simulink model "hw3"  (R2020b)
settings: Solver=FixedStepAuto  StartTime=0.0  StopTime=6  FixedStep=0.0001  RelTol=1e-3
model workspace (MAT data in the model file):
  Analog_Amplitude = 1
  Analog_Frequncy = 1
  period = 10
libraries: dsparch4 x1
settings Model: EnablePacing=on  Creator=max  LastModifiedBy=spraychamber

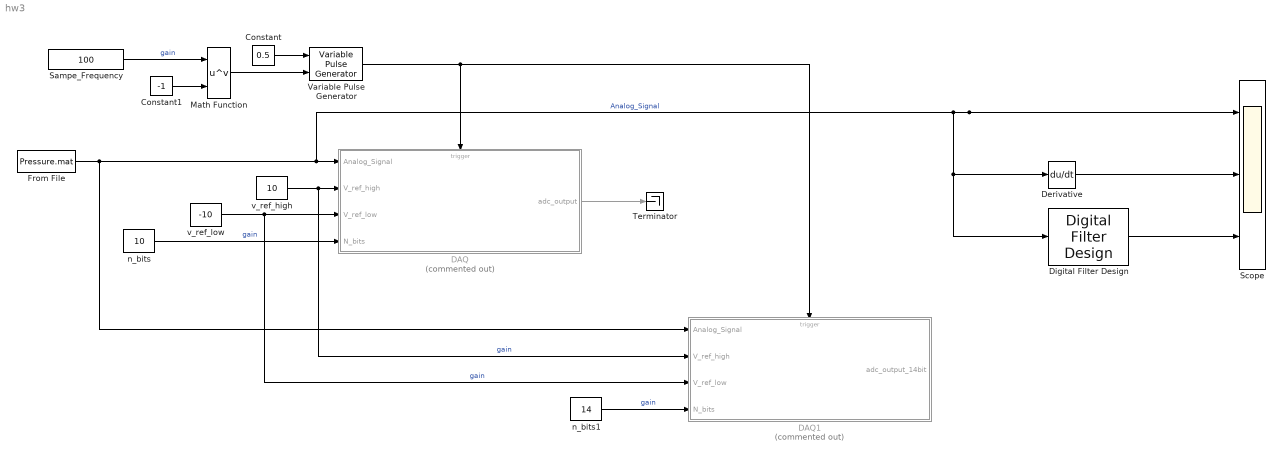
== system hw3 ==
  Constant : Constant  Value=0.5
  Constant1 : Constant  Value=-1
  DAQ : Subsystem  Commented=on
  DAQ1 : Subsystem  Commented=on
  Derivative : Derivative
  Digital Filter Design : dsparch4/Digital Filter Design  mwdsp_browser_bugfix_var=off
  From File : FromFile  FileName=Pressure.mat  ExtrapolationBeforeFirstDataPoint=Hold first value  InterpolationWithinTimeRange=Zero order hold  ExtrapolationAfterLastDataPoint=Hold last value
  Math Function : Math  Operator=pow  SaturateOnIntegerOverflow=on
  Sampe_Frequency : Constant  Value=100
  Scope : Scope  NumInputPorts=3
  Terminator : Terminator
  Variable Pulse Generator : VariablePulseGenerator  RunAtFixedTimeIntervals=on  SampleTime=0.0001
  n_bits : Constant  Value=10
  n_bits1 : Constant  Value=14
  v_ref_high : Constant  Value=10
  v_ref_low : Constant  Value=-10
  wires:
  From File/1 -> DAQ1/1(Analog_Signal), Digital Filter Design/1, Derivative/1, Scope/1, DAQ/1(Analog_Signal)  "Analog_Signal"
  Sampe_Frequency/1 -> Math Function/1  "gain"
  Constant/1 -> Variable Pulse Generator/1
  DAQ/1(adc_output) -> Terminator/1
  v_ref_low/1 -> DAQ1/3(V_ref_low), DAQ/3(V_ref_low)  "gain"
  v_ref_high/1 -> DAQ1/2(V_ref_high), DAQ/2(V_ref_high)  "gain"
  n_bits/1 -> DAQ/4(N_bits)  "gain"
  Variable Pulse Generator/1 -> DAQ1/Trigger, DAQ/Trigger
  Math Function/1 -> Variable Pulse Generator/2
  Constant1/1 -> Math Function/2
  n_bits1/1 -> DAQ1/4(N_bits)  "gain"
  Derivative/1 -> Scope/2
  Digital Filter Design/1 -> Scope/3

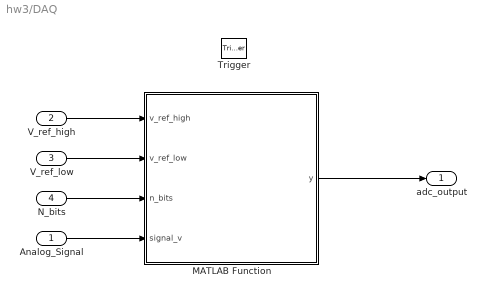
== system hw3/DAQ ==
  Analog_Signal : Inport
  V_ref_high : Inport  Port=2
  V_ref_low : Inport  Port=3
  N_bits : Inport  Port=4
  Trigger : TriggerPort  VariantControl=Variant  PortDimensions=1
  MATLAB Function : MATLAB Function  TreatAsAtomicUnit=on
  adc_output : Outport
  wires:
  V_ref_high/1 -> MATLAB Function/1(v_ref_high)
  V_ref_low/1 -> MATLAB Function/2(v_ref_low)
  Analog_Signal/1 -> MATLAB Function/4(signal_v)
  N_bits/1 -> MATLAB Function/3(n_bits)
  MATLAB Function/1(y) -> adc_output/1

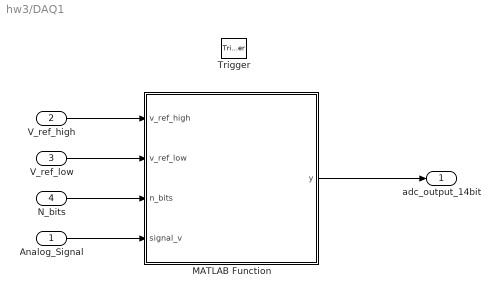
== system hw3/DAQ1 ==
  Analog_Signal : Inport
  V_ref_high : Inport  Port=2
  V_ref_low : Inport  Port=3
  N_bits : Inport  Port=4
  Trigger : TriggerPort  VariantControl=Variant  PortDimensions=1
  MATLAB Function : MATLAB Function  TreatAsAtomicUnit=on
  adc_output_14bit : Outport
  wires:
  V_ref_high/1 -> MATLAB Function/1(v_ref_high)
  V_ref_low/1 -> MATLAB Function/2(v_ref_low)
  Analog_Signal/1 -> MATLAB Function/4(signal_v)
  N_bits/1 -> MATLAB Function/3(n_bits)
  MATLAB Function/1(y) -> adc_output_14bit/1

== matlab function hw3/DAQ1/MATLAB Function ==
  data: v_ref_high input; y output; v_ref_low input; n_bits input; signal_v input
function y = daq(v_ref_high, v_ref_low, n_bits, signal_v)
v_ref_high = v_ref_high + abs(v_ref_low);
resolution = 2^n_bits;
delta = v_ref_high / resolution;
binary = zeros(resolution, 1);
signal_v = signal_v + abs(v_ref_low);
for i=1:resolution
    comparator = v_ref_high - (i - 1) * delta;
    bit = signal_v >= comparator;
    binary(i) = bit * comparator;
    if bit
        signal_v = signal_v - comparator;
    end
end
y = sum(binary) - abs(v_ref_low);

== matlab function hw3/DAQ/MATLAB Function ==
  data: v_ref_high input; y output; v_ref_low input; n_bits input; signal_v input
function y = daq(v_ref_high, v_ref_low, n_bits, signal_v)
v_ref_high = v_ref_high + abs(v_ref_low);
resolution = 2^n_bits;
delta = v_ref_high / resolution;
binary = zeros(resolution, 1);
signal_v = signal_v + abs(v_ref_low);
for i=1:resolution
    comparator = v_ref_high - (i - 1) * delta;
    bit = signal_v >= comparator;
    binary(i) = bit * comparator;
    if bit
        signal_v = signal_v - comparator;
    end
end
y = sum(binary) - abs(v_ref_low);
